simulink model "GreenCraneModel_LinearOrifices_test"  (R2024b)
settings: Solver=VariableStepAuto  StartTime=0.0  StopTime=20  RelTol=1e-5
model workspace (MATLAB code in the model file):
  | %% hydralic
  | %liqud data
  | rho_l = 850;
  | 
  | %Pressure
  | Ps = 110; %bar
  | 
  | %valve data
  | pRat = 30e5; %rated pressure
  | Cd = 0.6; %discarge coefficient
  | QRat = 270/6e4;
  | Admax = QRat/Cd/(2/rho_l*pRat/2)^0.5;
  | %% multibody
  | %Cylinder 1
  | sC_1 = 0.45; %Stroke
  | L0C_1 = 0.4; %Deadlength
  | x0C_1 = 0.05; %Initial position
  | dC_1 = 0.065; %Piston diameter
  | dRC_1 = 0.035; %Rod diameter
  | %Derived values
  | dOC_1 = dC_1 + dC_1/4; %Cylinder outer diameter
  | LC_1 = sC_1 + L0C_1/3; %Cylinder length
  | tEPC_1 = L0C_1/6; %Thickness of end plate
  | dJC_1 = L0C_1/3; %Diameter of joint
  | LJC_1 = dRC_1; %Length of joint
  | LRC_1 = sC_1 + tEPC_1; %Length of rod
  | tPC_1 = L0C_1/3; %Thickness of piston
  | AC_1 = pi*dC_1^2/4; %Piston area
  | ARC_1 = pi*dRC_1^2/4; %Rod area
  | AAC_1 = AC_1 - ARC_1; %Annulus area
  | Initial_Pos = x0C_1;
  | 
  | % crane arm
  | g=9.81;
  | theta1_init=0*pi/180;
  | thetaDot1_init=0;
  | L1=3.625;
  | rho=7800;
  | L4 = 0.229;
  | Lg4x = L1-L4/2;
  | Lg4y = 0.08157;
  | 
  | abx = 0.730-0.100-0.080; %0.550; %730-100-80
  | aby = (0.223-0.075); %-0.130; %0.223-75
  | g = 9.81;
  | G1 =100*g;
  | G4 = (4*76+16)*g;
  | 
  | G = 440*g; %440*g; %447.10945
  | Gx = 3.03499; %3.03499; %3.03499
  | Gy = 0.140; %0.2; %0.06071
  | 
  | Cy = -1.040;
  | Cx = 0.427;
  | ang_CA = atan2(Cy,Cx);
  | ang_k = atan2(aby,abx);
  | b = abs(sqrt(Cy^2+Cx^2));
  | c = abs(sqrt(abx^2+aby^2)); %56.73
  | % FBD Calculations
  | %syms Ax Ay P gamma beta ang_C ang_AB r_cb r_ab L3(i) w_A w_C VBx VBy Vp crs_abp
  | L3_min = 0.772;
  | L3 = L3_min+Initial_Pos; %0.5*(x-1)/(1000-1) + 0.772;  %.172*sin(X)/1 + 0.772+0.175 0;
  | 
  | ang_C = acos((L3^2+b^2-c^2)/(2*L3*b));
  | beta = ang_CA + pi - ang_C;
  | 
  | bx = L3*cos(beta) + Cx;
  | by = L3*sin(beta) + Cy;
  | ang_AB =atan2(by,bx);
  | gamma = ang_AB + ang_k;
  | 
  | r_cb = [L3*cos(beta);L3*sin(beta);0];
  | r_ab = [bx; by; 0 ];
  | 
  | 
  | crs_abp = cross(r_ab, [cos(beta); sin(beta);0]);
  | matrix = [1, 0, cos(beta);
  |           0, 1, sin(beta);
  |           0, 0, r_ab(1)*sin(beta) - r_ab(2)*cos(beta)];
  | right = [0;(G1+G4);G*(Gx*cos(gamma)-Gy*sin(gamma))];%(G1*cos(gamma)*L1/2+G4*(cos(gamma)*Lg4x-sin(gamma)*Lg4y))
  | 
  | ANS = inv(matrix)*right;
  | Ax = ANS(1);
  | Ay = ANS(2);
  | Fl  = ANS(3); %N
  | 
  | 
  | %% FF
  | dP_0 = 7e5; %Pressure drop with comp
  | phi = 0.7130;
  | A = AC_1; % Area piston side
  | Ar = AAC_1; % Area rod side
  | BW = 0; % deadband
  | SpoolTravel = 7; % Maximum Spool Travel
  | a = (SpoolTravel-BW)/25; % Valve Slope Characteristic [mm/(L/min)]
  | 
  | %deadband
  | DeadUp = 0.13;
  | DeadDown = 0.12;
  | 
  | %% Friction force from script
  |    F_friction = 1133.4; %N
  | 
  | %% Spool travel
  | 
  | 
  | 
  | % Down
  |     U_down_vec = [0, DeadDown ,0.2, 0.4, 0.6, 0.7, 0.8, 1.0];
  |     K_down = [1e-5,1e-5,0.75,2.17,3.39,3.99,4.55,4.84]/(6e4 * sqrt(1e5));
  |     Ad_down = (K_down/(Cd*sqrt(2/rho_l))) *1e6; %mm^2
  |     Ad_down2 = 1.5*Ad_down;
  |     Ad_max_PA =8.76; %mm^2
  |     Ad_max_BT = 1.2* Ad_max_PA;
  | 
  | 
  |     Ad_max_PB = 8.76; %mm^2
  |     Ad_max_AT = Ad_max_PB;
  | %     Dp_down_vec = [21.20, 32.96, 43.85, 48.10, 60.36]*1e5; %Pa pressure drop
  | %     VFR_down = [-3.55, -4.47, -5.18, -5.62, -6.191;
  | %            -9.95, -12.14, -14.83, -15.42, -18.60;
  | %            -14.10, -18.67, -22.17, -23.27, -27.33;
  | %            -16.96, -22.28, -27.57, -27.55, -33.1;
  | %            -17.88, -23.71, -29.04, -31.04, -35.92;
  | %            -20.53, -26.74, -32.73, -35.00, -37.53]/6e4; %m^3/s Flow
  | %     for i = 1:length(Dp_down_vec)
  | %         for j = 1:length(U_down_vec)
  | %         OAV_6x5 = sqrt( (VFR_down(i,j)).^2./(Cd^2*Dp_down_vec(i)*2/rho_l)  );
  | %         end
  | %     end
  | %
  | %
  | % % Up
  |     U_up_vec = [0, DeadUp ,0.2, 0.4, 0.6, 0.7, 0.8, 1.0];
  |     K_up = [1e-5,1e-5,0.78,2.29,3.42,4.59,5.09,5.71]/(6e4 * sqrt(1e5));
  |     Ad_up = (K_up/(Cd*sqrt(2/rho_l))) *1e6; %mm^2
  | %     Dp_up_vec = [17.39, 28.25, 36.01, 42.60, 56.50];
  | %     VFR_up = [3.36, 4.38, 4.90, 5.43, 5.86;
  | %               10.08, 12.24, 14.15, 15.51, 18.16;
  | %               9.25, 18.98, 22.92, 24.74, 27.65;
  | %               19.56, 24.95, 26.61, 29.47, 34.19;
  | %               14.84, 26.72, 32.17, 33.89, 38.51;
  | %               24.92, 26.56, 34.56, 38.50, 37.29];
  | %
  | 
  | %% motion ref
  | Amp = 0.1;
  | Mean = Amp;
values from neighbouring files (symbols this model uses):
  X = X_data.("<fPistonPosition_G_OPCfPistonPosition>")    [friksjon.m]
undefined symbols (not defined in the file or in its folder): Y, Z
libraries: sm_lib x35, fl_lib x31, nesl_utility x23, SimscapeFluids_lib x10, slpidlib x1
(part 3 of 3)

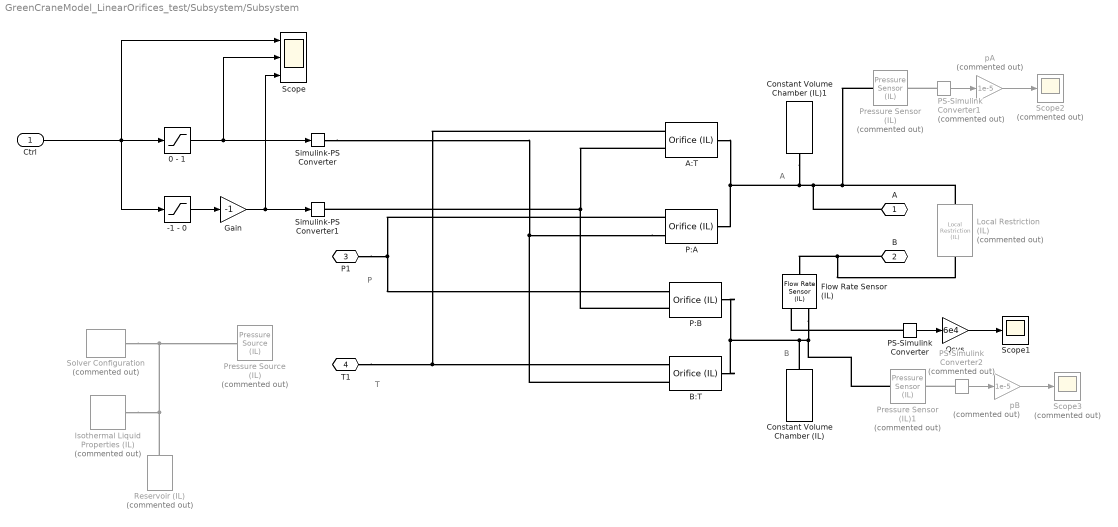
== system GreenCraneModel_LinearOrifices_test/Subsystem/Subsystem ==
  note: T
  note: B
  note: A
  note: P
  Ctrl : Inport
  -1 - 0 : Saturate  UpperLimit=0  LowerLimit=-1
  0 - 1 : Saturate  UpperLimit=1  LowerLimit=0
  A:T : SimscapeFluids_lib/Isothermal Liquid/Valves & Orifices/Orifices/Orifice (IL)  orifice_type=foundation.enum.constant_variable.variable  constant_orifice_spec=fluids.isothermal_liquid.valves_orifices.orifices.enum.constant_orifice_spec.area  variable_orifice_spec=fluids.isothermal_liquid.valves_orifices.orifices.enum.orifice_spec.linear  orifice_area_constant=1e-3 m^2  p_diff_TLU_constant=[-4, -3, -2, -1, -.5, 0, .5, 1, 2, 3, 4] MPa  vol_flow_TLU_constant=[-2.44, -2.12, -1.68, -1.22, -.84, 0, .85, 1.21, 1.7, 2.09, 2.41] .* 1e-3 m^3/s  S_min=0.12 m  del_S=0.88 m  open_orientation=fluids.isothermal_liquid.valves_orifices.orifices.enum.orifice_orientation.positive  area_max=1.8*Ad_max_AT mm^2  area_leak=0.1 mm^2  S_TLU=U_down_vec m  orifice_area_TLU=Ad_down mm^2  area=inf m^2  Cd=Cd  Re_c=150  smoothing_factor=0.01  pressure_recovery=false  S_vol_flow_TLU=[0, .002, .004, .007, .017] m  p_diff_TLU=[.3, .5, .7] MPa  vol_flow_TLU=1e-3 * [1.7e-05, 2e-05, 2.6e-05; .0035, .0045, .0053; .7, .9, 1.06; 1.96, 2.5, 3; 6, 7.7, 9.13] m^3/s
      settings: InternalSimscapePortConfiguration="{\"Bottom\":[],\"Left\":[{\"id\":\"A\",\"label\":\"A\",\"type\":\"foundation.isothermal_liquid.isothermal_liquid\"},{\"id\":\"S\",\"label\":\"S\",\"type\":\"input\"}],\"Right\":[{\"id\":\"B\",\"label\":\"B\",\"type\":\"foundation.isothermal_liquid.isothermal_liquid\"}],\"Top\":[]}"
  B:T : SimscapeFluids_lib/Isothermal Liquid/Valves & Orifices/Orifices/Orifice (IL)  orifice_type=foundation.enum.constant_variable.variable  constant_orifice_spec=fluids.isothermal_liquid.valves_orifices.orifices.enum.constant_orifice_spec.area  variable_orifice_spec=fluids.isothermal_liquid.valves_orifices.orifices.enum.orifice_spec.linear  orifice_area_constant=1e-3 m^2  p_diff_TLU_constant=[-4, -3, -2, -1, -.5, 0, .5, 1, 2, 3, 4] MPa  vol_flow_TLU_constant=[-2.44, -2.12, -1.68, -1.22, -.84, 0, .85, 1.21, 1.7, 2.09, 2.41] .* 1e-3 m^3/s  S_min=0.12 m  del_S=0.88 m  open_orientation=fluids.isothermal_liquid.valves_orifices.orifices.enum.orifice_orientation.positive  area_max=Ad_max_BT mm^2  area_leak=1e-10 m^2  S_TLU=U_down_vec m  orifice_area_TLU=Ad_down mm^2  area=inf m^2  Cd=Cd  Re_c=150  smoothing_factor=0.01  pressure_recovery=false  S_vol_flow_TLU=[0, .002, .004, .007, .017] m  p_diff_TLU=[.3, .5, .7] MPa  vol_flow_TLU=1e-3 * [1.7e-05, 2e-05, 2.6e-05; .0035, .0045, .0053; .7, .9, 1.06; 1.96, 2.5, 3; 6, 7.7, 9.13] m^3/s
      settings: InternalSimscapePortConfiguration="{\"Bottom\":[],\"Left\":[{\"id\":\"A\",\"label\":\"A\",\"type\":\"foundation.isothermal_liquid.isothermal_liquid\"},{\"id\":\"S\",\"label\":\"S\",\"type\":\"input\"}],\"Right\":[{\"id\":\"B\",\"label\":\"B\",\"type\":\"foundation.isothermal_liquid.isothermal_liquid\"}],\"Top\":[]}"
  Constant Volume Chamber (IL) : fl_lib/Isothermal Liquid/Elements/Constant Volume Chamber (IL)  volume=0.001 m^3  p_I_specify=off  p_I_priority=High  p_I=0.101325 MPa  p_I_nominal_specify=off  p_I_nominal_value=1  p_I_nominal_unit=MPa
      settings: InternalSimscapePortConfiguration="{\"Bottom\":[],\"Left\":[{\"id\":\"A\",\"label\":\"A\",\"type\":\"foundation.isothermal_liquid.isothermal_liquid\"}],\"Right\":[],\"Top\":[]}"
  Constant Volume Chamber (IL)1 : fl_lib/Isothermal Liquid/Elements/Constant Volume Chamber (IL)  volume=0.001 m^3  p_I_specify=off  p_I_priority=High  p_I=0.101325 MPa  p_I_nominal_specify=off  p_I_nominal_value=1  p_I_nominal_unit=MPa
      settings: InternalSimscapePortConfiguration="{\"Bottom\":[],\"Left\":[{\"id\":\"A\",\"label\":\"A\",\"type\":\"foundation.isothermal_liquid.isothermal_liquid\"}],\"Right\":[],\"Top\":[]}"
  Flow Rate Sensor (IL) : fl_lib/Isothermal Liquid/Sensors/Flow Rate Sensor (IL)  sensor_type=foundation.enum.mass_volumetric_sensor.volumetric
      settings: InternalSimscapePortConfiguration="{\"Bottom\":[],\"Left\":[{\"id\":\"A\",\"label\":\"A\",\"type\":\"foundation.isothermal_liquid.isothermal_liquid\"}],\"Right\":[{\"id\":\"B\",\"label\":\"B\",\"type\":\"foundation.isothermal_liquid.isothermal_liquid\"},{\"id\":\"V\",\"label\":\"V\",\"type\":\"output\"}],\"Top\":[]}"
  Gain : Gain  Gain=-1
  Isothermal Liquid Properties (IL) : fl_lib/Isothermal Liquid/Utilities/Isothermal Liquid Properties (IL)  Commented=on  rho_L_atm=998.21 kg/m^3  bulk_modulus_model=foundation.enum.bulk_modulus_model.const  beta_gain=6  beta_L_atm=2.1791e9 Pa  nu_atm=1.0034e-6 m^2/s  p_atm=0.101325 MPa  p_min=1 Pa  properties_range_check=simscape.enum.assert.action.error  air_fraction=0.005  polytropic_index=1.0  rho_g_atm=1.225 kg/m^3  air_dissolution_model=false  p_crit=3 MPa
  Local Restriction (IL) : fl_lib/Isothermal Liquid/Elements/Local Restriction (IL)  Commented=on  restriction_type=foundation.enum.restriction_type.fixed  restriction_area=10 mm^2  min_area=1e-10 m^2  max_area=0.005 m^2  area=inf m^2  Cd=0.64  Re_c=150  pressure_recovery=false
      settings: InternalSimscapePortConfiguration="{\"Bottom\":[],\"Left\":[{\"id\":\"A\",\"label\":\"A\",\"type\":\"foundation.isothermal_liquid.isothermal_liquid\"}],\"Right\":[{\"id\":\"B\",\"label\":\"B\",\"type\":\"foundation.isothermal_liquid.isothermal_liquid\"}],\"Top\":[]}"
  P:A : SimscapeFluids_lib/Isothermal Liquid/Valves & Orifices/Orifices/Orifice (IL)  orifice_type=foundation.enum.constant_variable.variable  constant_orifice_spec=fluids.isothermal_liquid.valves_orifices.orifices.enum.constant_orifice_spec.area  variable_orifice_spec=fluids.isothermal_liquid.valves_orifices.orifices.enum.orifice_spec.linear  orifice_area_constant=1e-3 m^2  p_diff_TLU_constant=[-4, -3, -2, -1, -.5, 0, .5, 1, 2, 3, 4] MPa  vol_flow_TLU_constant=[-2.44, -2.12, -1.68, -1.22, -.84, 0, .85, 1.21, 1.7, 2.09, 2.41] .* 1e-3 m^3/s  S_min=0.12 m  del_S=0.88 m  open_orientation=fluids.isothermal_liquid.valves_orifices.orifices.enum.orifice_orientation.positive  area_max=Ad_max_PA mm^2  area_leak=1e-10 m^2  S_TLU=U_down_vec m  orifice_area_TLU=Ad_down mm^2  area=inf m^2  Cd=Cd  Re_c=150  smoothing_factor=0.01  pressure_recovery=false  S_vol_flow_TLU=[0, .002, .004, .007, .017] m  p_diff_TLU=[.3, .5, .7] MPa  vol_flow_TLU=1e-3 * [1.7e-05, 2e-05, 2.6e-05; .0035, .0045, .0053; .7, .9, 1.06; 1.96, 2.5, 3; 6, 7.7, 9.13] m^3/s
      settings: InternalSimscapePortConfiguration="{\"Bottom\":[],\"Left\":[{\"id\":\"A\",\"label\":\"A\",\"type\":\"foundation.isothermal_liquid.isothermal_liquid\"},{\"id\":\"S\",\"label\":\"S\",\"type\":\"input\"}],\"Right\":[{\"id\":\"B\",\"label\":\"B\",\"type\":\"foundation.isothermal_liquid.isothermal_liquid\"}],\"Top\":[]}"
  P:B : SimscapeFluids_lib/Isothermal Liquid/Valves & Orifices/Orifices/Orifice (IL)  orifice_type=foundation.enum.constant_variable.variable  constant_orifice_spec=fluids.isothermal_liquid.valves_orifices.orifices.enum.constant_orifice_spec.area  variable_orifice_spec=fluids.isothermal_liquid.valves_orifices.orifices.enum.orifice_spec.linear  orifice_area_constant=1e-3 m^2  p_diff_TLU_constant=[-4, -3, -2, -1, -.5, 0, .5, 1, 2, 3, 4] MPa  vol_flow_TLU_constant=[-2.44, -2.12, -1.68, -1.22, -.84, 0, .85, 1.21, 1.7, 2.09, 2.41] .* 1e-3 m^3/s  S_min=0.12 m  del_S=0.88 m  open_orientation=fluids.isothermal_liquid.valves_orifices.orifices.enum.orifice_orientation.positive  area_max=Ad_max_PB mm^2  area_leak=0.1 mm^2  S_TLU=U_down_vec m  orifice_area_TLU=Ad_down mm^2  area=inf m^2  Cd=Cd  Re_c=150  smoothing_factor=0.01  pressure_recovery=false  S_vol_flow_TLU=[0, .002, .004, .007, .017] m  p_diff_TLU=[.3, .5, .7] MPa  vol_flow_TLU=1e-3 * [1.7e-05, 2e-05, 2.6e-05; .0035, .0045, .0053; .7, .9, 1.06; 1.96, 2.5, 3; 6, 7.7, 9.13] m^3/s
      settings: InternalSimscapePortConfiguration="{\"Bottom\":[],\"Left\":[{\"id\":\"A\",\"label\":\"A\",\"type\":\"foundation.isothermal_liquid.isothermal_liquid\"},{\"id\":\"S\",\"label\":\"S\",\"type\":\"input\"}],\"Right\":[{\"id\":\"B\",\"label\":\"B\",\"type\":\"foundation.isothermal_liquid.isothermal_liquid\"}],\"Top\":[]}"
  PS-Simulink Converter : nesl_utility/PS-Simulink Converter  PhysicalDomain=network_engine_domain  SubClassName=ps_output  LeftPortType=input  RightPortType=output  PseudoPeriodic=off  Frequencies=[]  VectorFormat=inherit  Unit=inherit  AffineConversion=off
  PS-Simulink Converter1 : nesl_utility/PS-Simulink Converter  Commented=on  PhysicalDomain=network_engine_domain  SubClassName=ps_output  LeftPortType=input  RightPortType=output  PseudoPeriodic=off  Frequencies=[]  VectorFormat=inherit  Unit=inherit  AffineConversion=off
  PS-Simulink Converter2 : nesl_utility/PS-Simulink Converter  Commented=on  PhysicalDomain=network_engine_domain  SubClassName=ps_output  LeftPortType=input  RightPortType=output  PseudoPeriodic=off  Frequencies=[]  VectorFormat=inherit  Unit=inherit  AffineConversion=off
  Pressure Sensor (IL) : fl_lib/Isothermal Liquid/Sensors/Pressure Sensor (IL)  Commented=on  pressure_measure=foundation.enum.pressure_measure.gauge
      settings: InternalSimscapePortConfiguration="{\"Bottom\":[],\"Left\":[{\"id\":\"A\",\"label\":\"A\",\"type\":\"foundation.isothermal_liquid.isothermal_liquid\"}],\"Right\":[{\"id\":\"Pg\",\"label\":\"Pg\",\"type\":\"output\"}],\"Top\":[]}"
  Pressure Sensor (IL)1 : fl_lib/Isothermal Liquid/Sensors/Pressure Sensor (IL)  Commented=on  pressure_measure=foundation.enum.pressure_measure.gauge
      settings: InternalSimscapePortConfiguration="{\"Bottom\":[],\"Left\":[{\"id\":\"A\",\"label\":\"A\",\"type\":\"foundation.isothermal_liquid.isothermal_liquid\"}],\"Right\":[{\"id\":\"Pg\",\"label\":\"Pg\",\"type\":\"output\"}],\"Top\":[]}"
  Pressure Source (IL) : fl_lib/Isothermal Liquid/Sources/Pressure Source (IL)  Commented=on  source_type=foundation.enum.constant_controlled.constant  pressure_differential=100 bar
      settings: InternalSimscapePortConfiguration="{\"Bottom\":[],\"Left\":[{\"id\":\"A\",\"label\":\"A\",\"type\":\"foundation.isothermal_liquid.isothermal_liquid\"}],\"Right\":[{\"id\":\"B\",\"label\":\"B\",\"type\":\"foundation.isothermal_liquid.isothermal_liquid\"}],\"Top\":[]}"
  Qsys : Gain  Gain=6e4
  Reservoir (IL) : fl_lib/Isothermal Liquid/Elements/Reservoir (IL)  Commented=on  reservoir_type=foundation.enum.constant_controlled.constant  pressure_spec=foundation.enum.pressure_spec.atmospheric  reservoir_pressure=0.101325 MPa
  Scope : Scope  NumInputPorts=3
  Scope1 : Scope
  Scope2 : Scope  Commented=on
  Scope3 : Scope  Commented=on
  Simulink-PS Converter : nesl_utility/Simulink-PS Converter  PhysicalDomain=network_engine_domain  SubClassName=ps_input  LeftPortType=input  RightPortType=output  PseudoPeriodic=off  Frequencies=[]  NoiseDistribution=none  NoiseParameters=[]  Unit=1  AffineConversion=off  FilteringAndDerivatives=filter  SimscapeFilterOrder=2  InputFilterTimeConstant=0.001  UdotUserProvided=0
  Simulink-PS Converter1 : nesl_utility/Simulink-PS Converter  PhysicalDomain=network_engine_domain  SubClassName=ps_input  LeftPortType=input  RightPortType=output  PseudoPeriodic=off  Frequencies=[]  NoiseDistribution=none  NoiseParameters=[]  Unit=1  AffineConversion=off  FilteringAndDerivatives=filter  SimscapeFilterOrder=2  InputFilterTimeConstant=0.001  UdotUserProvided=0
  Solver Configuration : nesl_utility/Solver Configuration  Commented=on  PhysicalDomain=network_engine_domain  SubClassName=solver  LeftPortType=input  RightPortType=generic  Tones=[]  Harmonics=[]  SimulateNoise=off  Profile=off  UseLocalSampling=off  EnableSwitchedLinearOptims=on  FrequencyDomain=off  UseCCode=off  RelTol=0.001  AbsTol=0.001  MinStep=1e-09  ToWorkspace=off  RevertToSquareIcSolve=off  NumHomotopyIterations=100  PhasorMode=off  PhasorModeNumHarmonics=1  ConsistencySolver=NEWTON_XTOL_AFTER_FTOL  IndexReductionMethod=DerivativeReplacement  DoDC=off  ResidualTolerance=1e-09  ConsistencyTolSource=GLOBAL  ConsistencyAbsTol=0.001  ConsistencyRelTol=0.001  ConsistencyTolFactor=0.001  UseLocalSolver=off  LocalSolverChoice=NE_BACKWARD_EULER_ADVANCER  ResolveIndetEquations=on  FunctionEvalNumThread=1  LocalSolverSampleTime=0.001  DoFixedCost=off  MaxNonlinIter=3  MaxModeIter=2  ComputeImpulses=off  ImpulseIterations=2  LinearAlgebra=auto  LinearAlgebraNumThread=0  EquationFormulation=NE_TIME_EF  DelaysMemoryBudget=1024  AutomaticFiltering=on  FilteringTimeConstant=0.001  PartitionStorageMethod=AS_NEEDED  PartitionMemoryBudget=1024  PartitionMethod=ROBUST  MultibodyUseLocalSolver=off  MultibodyLocalSolverChoice=ODE1  MultibodyLocalSolverSampleTime=0.001
  pA : Gain  Commented=on  Gain=1e-5
  pB : Gain  Commented=on  Gain=1e-5
  A : PMIOPort  Side=Left
  B : PMIOPort  Port=2  Side=Left
  P1 : PMIOPort  Port=3  Side=Right
  T1 : PMIOPort  Port=4  Side=Right
  wires:
  PS-Simulink Converter1/1 -> pA/1
  0 - 1/1 -> Scope/2, Simulink-PS Converter/1
  Qsys/1 -> Scope1/1
  PS-Simulink Converter/1 -> Qsys/1
  Ctrl/1 -> Scope/1, -1 - 0/1, 0 - 1/1
  Gain/1 -> Scope/3, Simulink-PS Converter1/1
  pB/1 -> Scope3/1
  -1 - 0/1 -> Gain/1
  pA/1 -> Scope2/1
  PS-Simulink Converter2/1 -> pB/1
  connections:
  A:T/LConn2 -- Simulink-PS Converter1/RConn1 -- P:B/LConn2
  A:T/RConn1 -- P:A/RConn1 -- A/RConn1 -- Pressure Sensor (IL)/LConn1 -- Local Restriction (IL)/LConn1 -- Constant Volume Chamber (IL)1/LConn1
  P:A/LConn2 -- Simulink-PS Converter/RConn1 -- B:T/LConn2
  P:A/LConn1 -- P1/RConn1 -- P:B/LConn1
  Isothermal Liquid Properties (IL)/RConn1 -- Reservoir (IL)/LConn1 -- Solver Configuration/RConn1 -- Pressure Source (IL)/LConn1
  Flow Rate Sensor (IL)/RConn1 -- Constant Volume Chamber (IL)/LConn1 -- B:T/RConn1 -- P:B/RConn1 -- Pressure Sensor (IL)1/LConn1
  PS-Simulink Converter/LConn1 -- Flow Rate Sensor (IL)/RConn2
  PS-Simulink Converter1/LConn1 -- Pressure Sensor (IL)/RConn1
  Local Restriction (IL)/RConn1 -- Flow Rate Sensor (IL)/LConn1 -- B/RConn1
  PS-Simulink Converter2/LConn1 -- Pressure Sensor (IL)1/RConn1
  A:T/LConn1 -- B:T/LConn1 -- T1/RConn1

== system GreenCraneModel_LinearOrifices_test/Subsystem/V_A ==
  Constant Volume Chamber (IL) : fl_lib/Isothermal Liquid/Elements/Constant Volume Chamber (IL)  volume=1 l  p_I_specify=off  p_I_priority=High  p_I=30 bar  p_I_nominal_specify=off  p_I_nominal_value=1  p_I_nominal_unit=MPa
      settings: InternalSimscapePortConfiguration="{\"Bottom\":[],\"Left\":[{\"id\":\"A\",\"label\":\"A\",\"type\":\"foundation.isothermal_liquid.isothermal_liquid\"}],\"Right\":[],\"Top\":[]}"
  Gain : Gain  Gain=1/10^5
  PS-Simulink Converter : nesl_utility/PS-Simulink Converter  PhysicalDomain=network_engine_domain  SubClassName=ps_output  LeftPortType=input  RightPortType=output  PseudoPeriodic=off  Frequencies=[]  VectorFormat=inherit  Unit=inherit  AffineConversion=off
  Pressure Sensor (IL) : fl_lib/Isothermal Liquid/Sensors/Pressure Sensor (IL)  pressure_measure=foundation.enum.pressure_measure.gauge
      settings: InternalSimscapePortConfiguration="{\"Bottom\":[],\"Left\":[{\"id\":\"A\",\"label\":\"A\",\"type\":\"foundation.isothermal_liquid.isothermal_liquid\"}],\"Right\":[{\"id\":\"Pg\",\"label\":\"Pg\",\"type\":\"output\"}],\"Top\":[]}"
  Connection Port : PMIOPort  Side=Left
  Out1 : Outport
  wires:
  Gain/1 -> Out1/1
  PS-Simulink Converter/1 -> Gain/1
  connections:
  Pressure Sensor (IL)/LConn1 -- Constant Volume Chamber (IL)/LConn1 -- Connection Port/RConn1
  PS-Simulink Converter/LConn1 -- Pressure Sensor (IL)/RConn1

== system GreenCraneModel_LinearOrifices_test/Subsystem/V_B ==
  Constant Volume Chamber (IL) : fl_lib/Isothermal Liquid/Elements/Constant Volume Chamber (IL)  volume=1 l  p_I_specify=off  p_I_priority=High  p_I=0.101325 MPa  p_I_nominal_specify=off  p_I_nominal_value=1  p_I_nominal_unit=MPa
      settings: InternalSimscapePortConfiguration="{\"Bottom\":[],\"Left\":[{\"id\":\"A\",\"label\":\"A\",\"type\":\"foundation.isothermal_liquid.isothermal_liquid\"}],\"Right\":[],\"Top\":[]}"
  Gain : Gain  Gain=1/10^5
  PS-Simulink Converter : nesl_utility/PS-Simulink Converter  PhysicalDomain=network_engine_domain  SubClassName=ps_output  LeftPortType=input  RightPortType=output  PseudoPeriodic=off  Frequencies=[]  VectorFormat=inherit  Unit=inherit  AffineConversion=off
  Pressure Sensor (IL) : fl_lib/Isothermal Liquid/Sensors/Pressure Sensor (IL)  pressure_measure=foundation.enum.pressure_measure.gauge
      settings: InternalSimscapePortConfiguration="{\"Bottom\":[],\"Left\":[{\"id\":\"A\",\"label\":\"A\",\"type\":\"foundation.isothermal_liquid.isothermal_liquid\"}],\"Right\":[{\"id\":\"Pg\",\"label\":\"Pg\",\"type\":\"output\"}],\"Top\":[]}"
  Connection Port : PMIOPort  Side=Left
  Out1 : Outport
  wires:
  Gain/1 -> Out1/1
  PS-Simulink Converter/1 -> Gain/1
  connections:
  Pressure Sensor (IL)/LConn1 -- Constant Volume Chamber (IL)/LConn1 -- Connection Port/RConn1
  PS-Simulink Converter/LConn1 -- Pressure Sensor (IL)/RConn1

== system GreenCraneModel_LinearOrifices_test/Subsystem/V_in ==
  Constant Volume Chamber (IL) : fl_lib/Isothermal Liquid/Elements/Constant Volume Chamber (IL)  volume=1 l  p_I_specify=on  p_I_priority=High  p_I=Ps bar  p_I_nominal_specify=off  p_I_nominal_value=1  p_I_nominal_unit=MPa
      settings: InternalSimscapePortConfiguration="{\"Bottom\":[],\"Left\":[{\"id\":\"A\",\"label\":\"A\",\"type\":\"foundation.isothermal_liquid.isothermal_liquid\"}],\"Right\":[],\"Top\":[]}"
  Gain : Gain  Gain=1/10^5
  PS-Simulink Converter : nesl_utility/PS-Simulink Converter  PhysicalDomain=network_engine_domain  SubClassName=ps_output  LeftPortType=input  RightPortType=output  PseudoPeriodic=off  Frequencies=[]  VectorFormat=inherit  Unit=inherit  AffineConversion=off
  Pressure Sensor (IL) : fl_lib/Isothermal Liquid/Sensors/Pressure Sensor (IL)  pressure_measure=foundation.enum.pressure_measure.gauge
      settings: InternalSimscapePortConfiguration="{\"Bottom\":[],\"Left\":[{\"id\":\"A\",\"label\":\"A\",\"type\":\"foundation.isothermal_liquid.isothermal_liquid\"}],\"Right\":[{\"id\":\"Pg\",\"label\":\"Pg\",\"type\":\"output\"}],\"Top\":[]}"
  Connection Port : PMIOPort  Side=Left
  Out1 : Outport
  wires:
  Gain/1 -> Out1/1
  PS-Simulink Converter/1 -> Gain/1
  connections:
  Pressure Sensor (IL)/LConn1 -- Constant Volume Chamber (IL)/LConn1 -- Connection Port/RConn1
  PS-Simulink Converter/LConn1 -- Pressure Sensor (IL)/RConn1

== system GreenCraneModel_LinearOrifices_test/Subsystem/p_0 ==
  In1 : Inport
  Gain : Gain  Gain=10^5
  Pressure Source (IL) : fl_lib/Isothermal Liquid/Sources/Pressure Source (IL)  source_type=foundation.enum.constant_controlled.controlled  pressure_differential=0 MPa
      settings: InternalSimscapePortConfiguration="{\"Bottom\":[],\"Left\":[{\"id\":\"A\",\"label\":\"A\",\"type\":\"foundation.isothermal_liquid.isothermal_liquid\"},{\"id\":\"P\",\"label\":\"P\",\"type\":\"input\"}],\"Right\":[{\"id\":\"B\",\"label\":\"B\",\"type\":\"foundation.isothermal_liquid.isothermal_liquid\"}],\"Top\":[]}"
  Reservoir (IL) : fl_lib/Isothermal Liquid/Elements/Reservoir (IL)  reservoir_type=foundation.enum.constant_controlled.constant  pressure_spec=foundation.enum.pressure_spec.atmospheric  reservoir_pressure=0.101325 MPa
  Simulink-PS Converter : nesl_utility/Simulink-PS Converter  PhysicalDomain=network_engine_domain  SubClassName=ps_input  LeftPortType=input  RightPortType=output  PseudoPeriodic=off  Frequencies=[]  NoiseDistribution=none  NoiseParameters=[]  Unit=1  AffineConversion=off  FilteringAndDerivatives=provide  SimscapeFilterOrder=1  InputFilterTimeConstant=0.001  UdotUserProvided=0
  Connection Port : PMIOPort  Side=Left
  wires:
  In1/1 -> Gain/1
  Gain/1 -> Simulink-PS Converter/1
  connections:
  Reservoir (IL)/LConn1 -- Pressure Source (IL)/LConn1
  Simulink-PS Converter/RConn1 -- Pressure Source (IL)/LConn2
  Connection Port/RConn1 -- Pressure Source (IL)/RConn1

== system GreenCraneModel_LinearOrifices_test/Subsystem1/V_A ==
  Constant Volume Chamber (IL) : fl_lib/Isothermal Liquid/Elements/Constant Volume Chamber (IL)  volume=1 l  p_I_specify=on  p_I_priority=High  p_I=68 bar  p_I_nominal_specify=off  p_I_nominal_value=1  p_I_nominal_unit=MPa
      settings: InternalSimscapePortConfiguration="{\"Bottom\":[],\"Left\":[{\"id\":\"A\",\"label\":\"A\",\"type\":\"foundation.isothermal_liquid.isothermal_liquid\"}],\"Right\":[],\"Top\":[]}"
  Gain : Gain  Gain=1/10^5
  PS-Simulink Converter : nesl_utility/PS-Simulink Converter  PhysicalDomain=network_engine_domain  SubClassName=ps_output  LeftPortType=input  RightPortType=output  PseudoPeriodic=off  Frequencies=[]  VectorFormat=inherit  Unit=inherit  AffineConversion=off
  Pressure Sensor (IL) : fl_lib/Isothermal Liquid/Sensors/Pressure Sensor (IL)  pressure_measure=foundation.enum.pressure_measure.gauge
      settings: InternalSimscapePortConfiguration="{\"Bottom\":[],\"Left\":[{\"id\":\"A\",\"label\":\"A\",\"type\":\"foundation.isothermal_liquid.isothermal_liquid\"}],\"Right\":[{\"id\":\"Pg\",\"label\":\"Pg\",\"type\":\"output\"}],\"Top\":[]}"
  Connection Port : PMIOPort  Side=Right
  Out1 : Outport
  wires:
  Gain/1 -> Out1/1
  PS-Simulink Converter/1 -> Gain/1
  connections:
  Pressure Sensor (IL)/LConn1 -- Constant Volume Chamber (IL)/LConn1 -- Connection Port/RConn1
  PS-Simulink Converter/LConn1 -- Pressure Sensor (IL)/RConn1

== matlab function GreenCraneModel_LinearOrifices_test/Subsystem1/CBV_opening ==
  data: pB input; uCBV output; pAm input; pA input
function uCBV = fcn(pB,pAm,pA)

pCr = 120;
alpha = 3;
dpopen = 100;
%uCBV = (alpha*pB + pAm - pCr - (alpha + 1)*pA)/dpopen;
uCBV = (alpha*pB + pAm - pCr)/dpopen; %vented
if uCBV < 0
    uCBV = 0;
elseif uCBV > 1
    uCBV = 1;
end

== matlab function GreenCraneModel_LinearOrifices_test/Subsystem/MATLAB Function1 ==
  data: pLS input; u output; pIn input
function u = fcn(pLS, pIn)

pCr = 7;
dp = 2;

u = (pLS + pCr - pIn)/dp;

if u < 0
    u = 0;
elseif u > 1
    u = 1;
end

== matlab function GreenCraneModel_LinearOrifices_test/Subsystem2/hastighets profil ==
  data: y output; t input
function y  = fcn(t)
v_max = 0.1;
v_0 = 0;
x_0 = 0;
x_max = 0.05;
x_max = 0.25;
t_ramp = 1;
v_ref = x_max/t_ramp;
start_time = 1;
hold_time = 1;
if v_ref>v_max
    v_ref=v_max;
    y=0;
end
t1 = start_time;
t2 = t1 + t_ramp;
t3 = t2 + hold_time;
t4 = t3 + t_ramp; 
t5 = t4 + start_time;
t6 = t5 + t_ramp;
t7 = t6 + hold_time;
t8 = t7 + t_ramp;
t9 = t8 + start_time;
if t < t1
    y = x_0;
elseif t < t2 % ramp up speed
    y = x_0 + v_0*(t-t1) + v_ref*(t-t1);
elseif t < t3 %holding speed
    y = x_0 + v_ref*t_ramp;
elseif t < t4 %ramping down speed
    y = x_0 + v_ref*t_ramp - v_ref*(t-t3);
elseif t < t5 %holding 0
    y = x_0;

elseif t < t6 %ramping down speed
    y = x_0 - v_0*(t-t5) - v_ref*(t-t5);
elseif t < t7 %holdin speed
    y = x_0 - v_ref*t_ramp;
elseif t < t8 %ramping up speed
    y = x_0 - v_ref*t_ramp + v_ref*(t-t7);
elseif t < t9 %holding 0
    y = x_0;
end

== matlab function GreenCraneModel_LinearOrifices_test/CTRL/V2Q2u ==
  data: Ps input; Pa input; Pb input; x_dot input; u output; dP output; A parameter; Ar parameter; Q_lm output; DeadUp parameter; DeadDown parameter
function [u, dP,Q_lm] =fcn(Ps, Pa, Pb, x_dot, A, Ar,DeadUp, DeadDown)
% if x_dot > 0
%     Q = x_dot * A; % Wantedlow
%     dP = (Ps-Pa)*1e5;
%     dp_ref = abs(dP_0/dP);
%     %dp_ref = 1;
%     Q_star = (Q * sqrt(dp_ref)) * 6e4; % Referancelow [L/min]
%     u = (Q_star * a + BW)/SpoolTravel; % Control Signal [-1, 1]
% 
% elseif x_dot < 0
%     Q = x_dot * (A*phi); % Wantedlow
%     dP = (Ps-Pb)*1e5;
%     dp_ref = abs(dP_0/dP);
%    % dp_ref = 1;
%     Q_star = (Q * sqrt(dp_ref)) * 6e4; % Referancelow [L/min]
%     u = (Q_star * a - BW)/SpoolTravel; % Control Signal [-1, 1]
% 
% else
%     Q_star = 0;
%     dP = 0;
%     u = 0;
% 
% end
% Q_lm = Q_star; %Q * 6e4;
% end

%Kref
	K02Up = 0.78; 
	K04Up = 2.29; 
	K06Up = 3.42;
	K07Up = 4.59; 
	K08Up = 5.09; 
	K1Up = 5.71; 
	
	K02Down = -0.75; 
	K04Down = -2.17; 
	K06Down = -3.39; 
	K07Down = -3.99; 
	K08Down = -4.55;
	K1Down = -4.84; 

Q_lm =0;
dP = Ps-Pa;
if x_dot >= 0.0  % Upwards
    Q_lm = A * x_dot * 6e4;
	dP = Ps-Pa;
    if dP < 0
    dP = 1;
    end
	KRef = Q_lm / sqrt(dP) ;
	if KRef < 0.0 
		UTemp = 0.0;
    elseif KRef <K02Up 
		UTemp = -KRef/K02Up * (0.2 - DeadUp);
    elseif KRef <K04Up 
		UTemp = -(0.2 -DeadUp) -( KRef-K02Up)/(K04Up-K02Up) * (0.4-DeadUp-0.2);
    elseif KRef <K06Up 
		UTemp = -(0.4 -DeadUp-0.2) -(0.2 -DeadUp)  -(KRef-K04Up)/(K06Up-K04Up) * (0.6-DeadUp-0.4);
    elseif KRef <K07Up 
		UTemp = -(0.6 -DeadUp-0.4) -(0.4 -DeadUp-0.2) -(0.2 -DeadUp) -(KRef-K06Up)/(K07Up-K06Up) * (0.7-DeadUp-0.6);
    elseif KRef <K08Up 
		UTemp = -(0.7 -DeadUp-0.6) -(0.6 -DeadUp-0.4) -(0.4 -DeadUp-0.2) -(0.2 -DeadUp) -(KRef-K07Up)/(K08Up-K07Up) * (0.8-DeadUp-0.7);
    elseif KRef <K1Up 
		UTemp = -(0.8 -DeadUp-0.7) -(0.7 -DeadUp-0.6) -(0.6 -DeadUp-0.4) -(0.4 -DeadUp-0.2) -(0.2 -DeadUp) -(KRef-K08Up)/(K1Up-K08Up) * (1.0-DeadUp-0.8);
    else
		UTemp = -(1-DeadUp);
    end

elseif x_dot < 0.0 % Downwards
	
	Q_lm =Ar *x_dot * 6e4;
	dP =Ps-Pb;
    if dP < 0
        dP = 1;
    end
	KRef = Q_lm / sqrt(dP);
	
if KRef > 0.0 
	    UTemp = 0.0;
    elseif KRef >K02Down 
		UTemp =KRef/K02Down * (0.2-DeadDown);
    elseif KRef >K04Down 
		UTemp = (0.2 -DeadDown) + (KRef-K02Down)/(K04Down-K02Down) * (0.4 -DeadDown - 0.2);
    elseif KRef >K06Down 
		UTemp = (0.4 -DeadDown - 0.2)+(0.2 -DeadDown) + (KRef-K04Down)/(K06Down-K04Down) * (0.6 -DeadDown - 0.4);
    elseif KRef >K07Down 
		UTemp = (0.6 -DeadDown - 0.4)+(0.4 -DeadDown - 0.2)+(0.2 -DeadDown) + (KRef-K06Down)/(K07Down-K06Down) * (0.7 -DeadDown - 0.6);
    elseif KRef >K08Down 
		UTemp = (0.7 -DeadDown - 0.6)+(0.6 -DeadDown - 0.4)+(0.4 -DeadDown - 0.2)+(0.2 -DeadDown) + (KRef-K07Down)/(K08Down-K07Down) * (0.8 -DeadDown - 0.7);
    elseif KRef >K1Down 
		UTemp = (0.8 -DeadDown-0.7)+(0.7 -DeadDown - 0.6)+(0.6 -DeadDown - 0.4)+(0.4 -DeadDown - 0.2)+(0.2 -DeadDown) + (KRef-K08Down)/(K1Down-K08Down) * (1.0 -DeadDown - 0.8);
    else
		UTemp = (1.0-DeadDown);
    end
else
    UTemp = 0;
end
u = UTemp;

== matlab function GreenCraneModel_LinearOrifices_test/Subsystem/MATLAB Function ==
  data: u input; pLS output; pA input; pB input
function pLS = fcn(u,pA,pB)
uEps = 0.05; %Deadband
if u < -uEps
    pLS = pB;
elseif u < uEps
    pLS = 0;
else
    pLS = pA;
end

== matlab function GreenCraneModel_LinearOrifices_test/CTRL/MATLAB Function ==
  data: u input; u_PID input; U output; DeadDown parameter; DeadUp parameter
function U = fcn(u,u_PID, DeadDown, DeadUp)
u_ref = u-u_PID;
if u_ref >0
    U = u_ref+DeadDown;
elseif u_ref < 0
     U = u_ref-DeadUp;
else 
     U = 0;
end

== matlab function GreenCraneModel_LinearOrifices_test/Subsystem2/MATLAB Function1 ==
  data: cosine input; ramp_vel input; sine input; ramp_pos input; xRef output; enable input; xDotRef output
function [xRef, xDotRef] = fcn(cosine, ramp_vel,sine, ramp_pos, enable)
if enable == 1    
    xRef = sine;
else
    xRef = ramp_pos;
end

if enable == 1    
    xDotRef = cosine;
else
    xDotRef = ramp_vel;
end
